simulink model "TEST"  (R2022b)
settings: Solver=VariableStepAuto  StartTime=0.0  StopTime=10.0  RelTol=1e-3
settings Model: Creator=Ccm  LastModifiedBy=Ccm

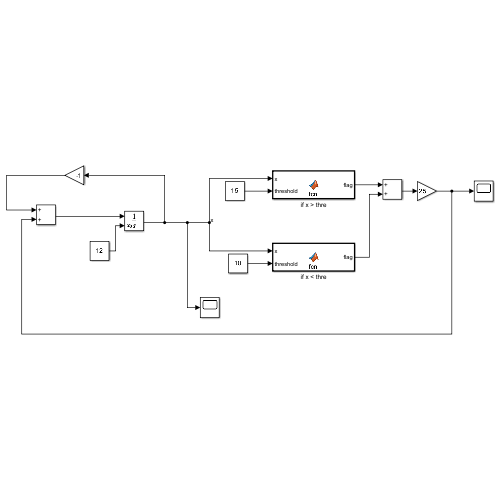
[thumbnail: Simulink's stored preview of the top-level diagram]
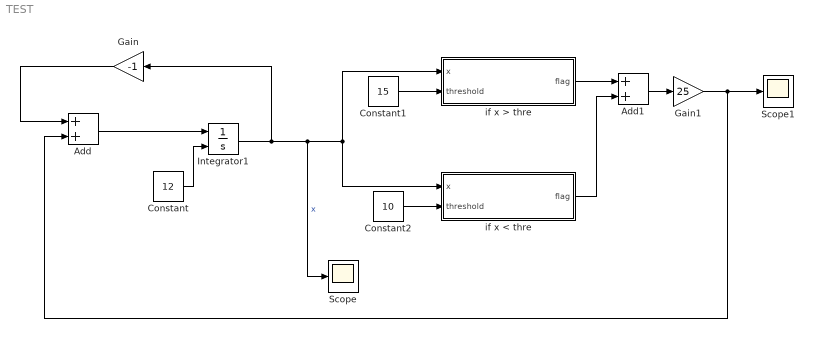
== system TEST ==
  Add : Sum
  Add1 : Sum
  Constant : Constant  Value=12
  Constant1 : Constant  Value=15
  Constant2 : Constant  Value=10
  Gain : Gain  Gain=-1
  Gain1 : Gain  Gain=25
  Integrator1 : Integrator  InitialConditionSource=external
  Scope : Scope
  Scope1 : Scope
  if x < thre : MATLAB Function  TreatAsAtomicUnit=on
  if x > thre : MATLAB Function  TreatAsAtomicUnit=on
  wires:
  Integrator1/1 -> Scope/1, if x > thre/1(x), if x < thre/1(x), Gain/1  "x"
  Constant/1 -> Integrator1/2
  Gain1/1 -> Scope1/1, Add/2
  Gain/1 -> Add/1
  Add/1 -> Integrator1/1
  Add1/1 -> Gain1/1
  if x > thre/1(flag) -> Add1/1
  if x < thre/1(flag) -> Add1/2
  Constant1/1 -> if x > thre/2(threshold)
  Constant2/1 -> if x < thre/2(threshold)

== matlab function TEST/if x > thre ==
  data: x input; flag output; threshold input
function flag= fcn(x,threshold)

if x > threshold
    flag = 1;
else
    flag =0 ;
end

== matlab function TEST/if x < thre ==
  data: x input; flag output; threshold input
function flag = fcn(x,threshold)

if x < threshold
    flag = 1;
else
    flag = 0;
end
